simulink model "ShubhamGupta_180749_Lab6_P"  (R2020b)
settings: Solver=VariableStepAuto  StartTime=0.0  StopTime=100  RelTol=1e-3
settings Model: Creator=sampadasinha  LastModifiedBy=subhamgupta
settings DataIOCC: ReturnWorkspaceOutputs=off

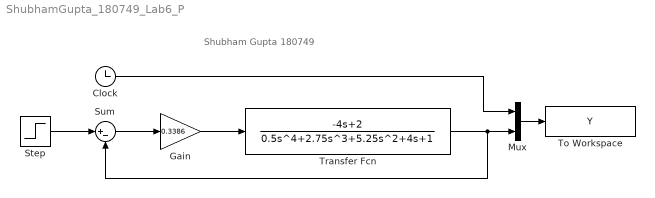
== system ShubhamGupta_180749_Lab6_P ==
  note: Shubham Gupta 180749
  Clock : Clock
  Gain : Gain  Gain=0.3386
  Mux : Mux  Inputs=2
  Step : Step  Time=0  SampleTime=0
  Sum : Sum  Inputs=|+-
  To Workspace : ToWorkspace  VariableName=Y  SampleTime=-1
  Transfer Fcn : TransferFcn  Numerator=[-4 2]  Denominator=[0.5 2.75 5.25 4 1]
  wires:
  Sum/1 -> Gain/1
  Step/1 -> Sum/1
  Transfer Fcn/1 -> Sum/2, Mux/2
  Gain/1 -> Transfer Fcn/1
  Mux/1 -> To Workspace/1
  Clock/1 -> Mux/1
